simulink model "asbQuadcopters"  (Simulink 9.1)
settings: Solver=VariableStepAuto  StartTime=0.0  StopTime=TFinal  RelTol=1e-3
values from neighbouring files (symbols this model uses):
  Controller =     [data_set.mat]
  Estimator =     [data_set.mat]
  g = 9.81    [data_set.mat]
  init =     [data_set.mat]
  Sensors =     [data_set.mat]
  takeOffDuration = 1    [data_set.mat]
  Ts = 0.005    [data_set.mat]
  Vehicle =     [data_set.mat]
undefined symbols (not defined in the file or in its folder): DiscIntNeverNeededParam, Discrete, Earth, ft, m, s, sigbuilder_block, Time, WGS84
libraries: simulink x39, aerolibconvert2 x4, ctrlSharedLib x3, sharedtransform x3, aerolibfltsims x2, aerolibutil x2, shared6dof x1, aerolibasang x1, dynamicsLibrary x1, aerolibtransform2 x1, environmentLibrary x1, sharedutil x1
(part 1 of 3)
settings Model: SuppressorTable="22 serialization::archive 11 0 6 0 0 1 8 0 0 0 0 6 0 0 1 0 39 asbQuadcopters/Command/Live Time  Ticks 0 6 0 0 2 8 0 0 0 0 6 41 Simulink:DataType:WarningOverFlowDetected 0 0 0 6 0  0  0 0 0 0 8 20160523 0 0 0 10 57 55 0 1 40 SimulinkFixedPoint:util:Overflowoccurred 0 0 0  0  8 20160523 0 10 57 55 0 1"  LogicAnalyzerSignalOrdering=2e0c0a72-345e-4dc5-9c0e-29032ec30a1e,a96d9f9d-3ef5-4050-b6b8-b8019fd01667,c8d366ad-4d1f-40bd-a54a-09e26b883270,8941bdc4-4fa0-4569-8040-854ce7cb60c2,e7686d44-45c9-4c55-ba5d-06b91bc522a8,a75aae3c-0a7a-4dbc-8a75-97ed30805da8,7c481f21-a942-450d-9b23-3950506eae04,f4ffd508-2ff6-4be3-84ec-4b50dbf29143,1f3924a1-458c-46a2-8b2c-9c14621b8789,e4a67875-028c-4c14-9c8e-409b915de7ac  Creator=DES  LastModifiedBy=DES
settings DataIOCC: SaveFormat=Dataset
settings OptimizationCC: LifeSpan=auto
settings DebuggingCC: UnderspecifiedInitializationDetection=Simplified  MergeDetectMultiDrivingBlocksExec=error  SFUnexpectedBacktrackingDiag=error  SFNoUnconditionalDefaultTransitionDiag=error  SFExecutionAtInitializationDiag=warning
settings HardwareCC: ProdBitPerPointer=64  ProdBitPerSizeT=64  ProdBitPerPtrDiffT=64  ProdLargestAtomicFloat=Float  ProdIntDivRoundTo=Zero  ProdEndianess=LittleEndian  ProdWordSize=64  ProdHWDeviceType=Intel->x86-64 (Windows64)
settings ModelReferenceCC: PropagateSignalLabelsOutOfModel=on
settings CodeAppCC: StateflowObjectComments=off
settings GRTTargetCC: TargetLangStandard=C99 (ISO)  CombineOutputUpdateFcns=on  GRTInterface=off
settings ConfigComp: CovMetricSettings=dwe  CovHtmlReporting=off  CovSaveCumulativeToWorkspaceVar=off  CovSaveSingleToWorkspaceVar=off  CovExternalEMLEnable=on

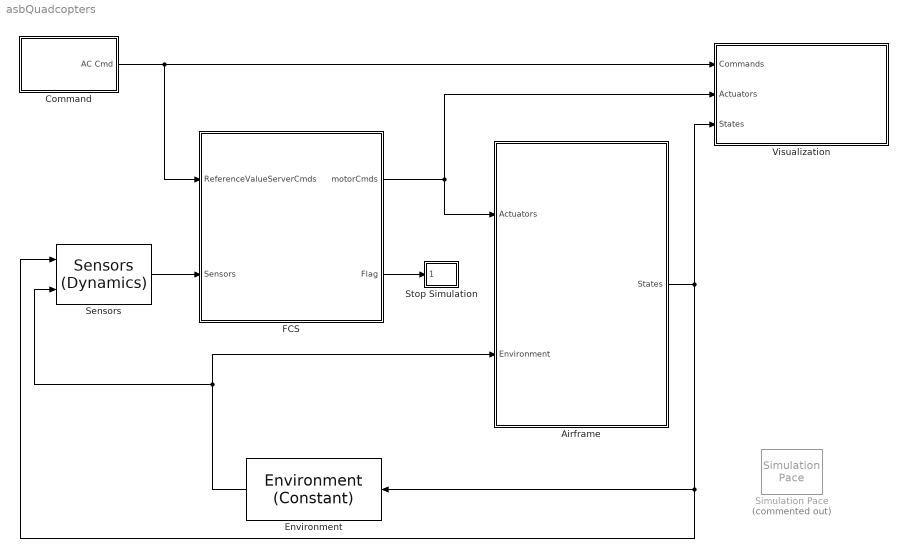
== system asbQuadcopters ==
  Airframe : Subsystem  TreatAsAtomicUnit=on
  Command : Subsystem
  "Environment " : environmentLibrary/Environment (Constant)  VariantControl=VSS_ENVIRONMENT_CST
      settings: SourceProductName=Aerospace Blockset  SourceProductBaseCode=AE
  FCS : Subsystem
  Sensors : sensorsLibrary/Sensors (Dynamics)  SystemSampleTime=-1  VariantControl=VSS_SENSORS_DYNAMICS
      settings: SourceProductName=Aerospace Blockset  SourceProductBaseCode=AE
  Simulation Pace : aerolibanimutils/Simulation Pace  Commented=on  SimulationPace=1  SleepMode=MATLAB Thread  OutputPaceError=off  SampleTime=Ts
      settings: AttributesFormatString=%<SimulationPace> sec/sec
  Stop Simulation : Subsystem
  Visualization : Subsystem
  wires:
  Command/1(AC Cmd) -> Visualization/1(Commands), FCS/1(ReferenceValueServerCmds)
  Sensors/1 -> FCS/2(Sensors)
  Airframe/1(States) -> Visualization/3(States), Sensors/1, "Environment "/1
  "Environment "/1 -> Sensors/2, Airframe/2(Environment)
  FCS/2(Flag) -> Stop Simulation/1(Flags)
  FCS/1(motorCmds) -> Visualization/2(Actuators), Airframe/1(Actuators)

== system asbQuadcopters/Airframe ==
  Actuators : Inport
  Environment : Inport  Port=2
  6DOF (Quaternion) : shared6dof/6DOF (Euler Angles)  units=Metric (MKS)  mtype=Fixed  rep=Euler Angles  xme_0=init.posNED  Vm_0=init.vb  eul_0=init.euler  pm_0=init.angRates  mass_0=Vehicle.Airframe.mass  mass_e=0.5  mass_f=2.0  inertia=Vehicle.Airframe.inertia  inertia_e=eye(3)  inertia_f=2*eye(3)  k_quat=Vehicle.SixDOF.quatGain  vre_flag=on  abi_flag=on  aMode=aMode
      settings: SourceProductBaseCode=AE
  AC model : Subsystem
  Bus setup : Subsystem
  Position on Earth : Subsystem  Priority=1  TreatAsAtomicUnit=on
  Terminator : Terminator
  States : Outport
  wires:
  Actuators/1 -> AC model/1(Actuators)
  Environment/1 -> AC model/2(Environment)
  AC model/1(F_cg) -> 6DOF (Quaternion)/1
  AC model/2(M_cg) -> 6DOF (Quaternion)/2
  6DOF (Quaternion)/1 -> Bus setup/2(V_ned)
  6DOF (Quaternion)/2 -> Position on Earth/1(Xe), Bus setup/3(X_ned)
  6DOF (Quaternion)/3 -> Bus setup/4(Euler)
  6DOF (Quaternion)/6 -> AC model/5(w_b), Bus setup/7(Omega_b)
  6DOF (Quaternion)/7 -> Bus setup/8(dOmega_b)
  6DOF (Quaternion)/9 -> Bus setup/9(Accel_b)
  Bus setup/1(States) -> States/1
  Position on Earth/1(LLA) -> Bus setup/1(LLA)
  6DOF (Quaternion)/5 -> AC model/4(V_b), Bus setup/6(V_b)
  6DOF (Quaternion)/4 -> AC model/3(DCM_be), Bus setup/5(DCM_be)
  6DOF (Quaternion)/8 -> Terminator/1

== system asbQuadcopters/Command ==
  Bus Creator : BusCreator  Inputs=5  OutDataTypeStr=Bus: CommandBus  NonVirtualBus=on
  Clock : Clock
  Compare To Constant : simulink/Logic and Bit Operations/Compare To Constant  relop=<  const=takeOffDuration  OutDataTypeStr=boolean
  Compare To Zero : simulink/Logic and Bit Operations/Compare To Zero  relop===  OutDataTypeStr=boolean
  Compare To Zero1 : simulink/Logic and Bit Operations/Compare To Zero  relop===  OutDataTypeStr=boolean
  Data Type Conversion1 : DataTypeConversion  OutDataTypeStr=single
  Data Type Conversion3 : DataTypeConversion  OutDataTypeStr=single
  Live Time  Ticks : simulink/Sources/Counter Free-Running  NumBits=32  tsamp=Ts
  Logical Operator : Logic  AllPortsSameDT=off  OutDataTypeStr=boolean
  Mux : Mux  Inputs=3
  Mux1 : Mux  Inputs=3
  Position/Attitude Reference : Subsystem  Tag=STV Subsys  LoadFcn=sigbuilder_block('load');  StartFcn=sigbuilder_block('start');  StopFcn=sigbuilder_block('stop');  ClipboardFcn=sigbuilder_block('clipboard');  mask(Sigbuilder block){tuvar=[0:10]}
      mask help: Simulink:masks:SigbuilderBlock_MD
      mask init:
      | if ~strcmp(get_param(bdroot(gcbh),'SimulationStatus'),'stopped') tuvar = sigbuilder_block('maskInit'); end
      settings: CopyFcn=sigbuilder_block('copy');  DeleteFcn=sigbuilder_block('delete');  ModelCloseFcn=sigbuilder_block('modelClose');  PreSaveFcn=sigbuilder_block('preSave');  PauseFcn=sigbuilder_block('pause');  ContinueFcn=sigbuilder_block('continue');  NameChangeFcn=sigbuilder_block('namechange');  OpenFcn=sigbuilder_block('open',[-738.75 224.25 556.5 329.25 ]);  CloseFcn=sigbuilder_block('close');
      mask Display: plot(0, 0, 100, 100,[2, 2, 32, 32, 2], [68, 8, 8, 68, 68],[32, 2], [38, 38], [32, 19, 2],[53, 60, 44], [32, 17, 17, 2],[16, 16, 31, 31]);txt = getActiveGroup(gcbh);text(2, 100, txt,'verticalAlignment', 'top');
  Rate Transition{1..4} (4 alike) : RateTransition  OutPortSampleTime=Ts
  AC Cmd : Outport  OutDataTypeStr=Bus: CommandBus
  wires:
  Bus Creator/1 -> AC Cmd/1
  Position/Attitude Reference/3(Z) -> Mux1/3
  Live Time  Ticks/1 -> Bus Creator/5  "live_time_ticks"
  Position/Attitude Reference/6(Roll) -> Compare To Zero/1, Mux/3  "roll_cmd"
  Position/Attitude Reference/5(Pitch) -> Mux/2, Compare To Zero1/1  "pitch_cmd"
  Compare To Zero1/1 -> Logical Operator/2
  Rate Transition4/1 -> Bus Creator/1  "controlModePosVSOrient"
  Position/Attitude Reference/2(Y) -> Mux1/2
  Rate Transition3/1 -> Bus Creator/3  "takeoff_flag"
  Position/Attitude Reference/4(Yaw) -> Mux/1  "yaw_cmd"
  Data Type Conversion1/1 -> Rate Transition2/1
  Compare To Zero/1 -> Logical Operator/1
  Logical Operator/1 -> Rate Transition4/1
  Mux1/1 -> Data Type Conversion1/1
  Mux/1 -> Data Type Conversion3/1
  Rate Transition2/1 -> Bus Creator/2  "pos_ref"
  Data Type Conversion3/1 -> Rate Transition1/1
  Compare To Constant/1 -> Rate Transition3/1
  Clock/1 -> Compare To Constant/1
  Rate Transition1/1 -> Bus Creator/4  "orient_ref"
  Position/Attitude Reference/1(X) -> Mux1/1

== system asbQuadcopters/FCS ==
  note: Derived from the work by Sertac
      | Karaman and Fabian Riether
  ReferenceValueServerCmds : Inport  OutDataTypeStr=Bus: CommandBus
  Sensors : Inport  Port=2  OutDataTypeStr=Bus: SensorsBus  BusOutputAsStruct=on
  Bus Selector : BusSelector  OutputSignals=controlModePosVSOrient
  Bus Selector1 : BusSelector  OutputSignals=usePosVIS_flag,opticalFlow_data,posVIS_data
  Bus Selector2 : BusSelector  OutputSignals=HAL_acc_SI,HAL_gyro_SI,HAL_ultrasound_SI,HAL_pressure_SI,HAL_vbat_SI
  Bus Selector3 : BusSelector  OutputSignals=HALSensors
  Bus Selector4 : BusSelector  OutputSignals=VisionSensors,SensorCalibration
  Crash Predictor Flags : Subsystem
  Logging : Subsystem  TreatAsAtomicUnit=on
      settings: RTWFcnNameOpts=Use subsystem name
  ReferenceValueServerCmds_1 : InportShadow  OutDataTypeStr=Bus: CommandBus
  Sensors_1 : InportShadow  Port=2  OutDataTypeStr=Bus: SensorsBus  BusOutputAsStruct=on
  Sensors_2 : InportShadow  Port=2  OutDataTypeStr=Bus: SensorsBus  BusOutputAsStruct=on
  State Estimator : Subsystem
  controller : Subsystem
  sensordata_group : Subsystem
  motorCmds : Outport
  Flag : Outport  Port=2
  wires:
  Bus Selector4/2 -> State Estimator/6(sensorCalibration_datin)  "<SensorCalibration>"
  Bus Selector3/1 -> Bus Selector2/1  "<HALSensors>"
  Bus Selector1/3 -> State Estimator/5(posVIS_datin)  "<posVIS_data>"
  Bus Selector/1 -> State Estimator/1(controlModePosVSOrient_flagin)  "<controlModePosVSOrient>"
  Bus Selector2/1 -> sensordata_group/1(HAL_acc_SI)  "<HAL_acc_SI>"
  State Estimator/1(states_estim) -> controller/2(states_estim), Crash Predictor Flags/1(states_estim), Logging/3(states_estim)
  controller/1(motors_refout) -> motorCmds/1, Logging/1(motorCmds)
  Bus Selector2/4 -> sensordata_group/4(HAL_pressure_SI)  "<HAL_pressure_SI>"
  Bus Selector1/1 -> State Estimator/3(usePosVIS_flagin)  "<usePosVIS_flag>"
  sensordata_group/1(sensordata_datin) -> State Estimator/2(sensor_data_in), Logging/6(sensordata_datin)
  Bus Selector1/2 -> State Estimator/4(opticalFlow_datin)  "<opticalFlow_data>"
  ReferenceValueServerCmds/1 -> controller/1(ReferenceValueServerBus), Bus Selector/1
  controller/2(pose_refout) -> Logging/2(posRef)
  Bus Selector4/1 -> Bus Selector1/1  "<VisionSensors>"
  Sensors_1/1 -> Crash Predictor Flags/2(Sensors), Bus Selector4/1
  Bus Selector2/2 -> sensordata_group/2(HAL_gyro_SI)  "<HAL_gyro_SI>"
  Bus Selector2/3 -> sensordata_group/3(HAL_ultrasound_SI)  "<HAL_ultrasound_SI>"
  Sensors/1 -> Bus Selector3/1
  Crash Predictor Flags/1(Flag) -> Flag/1
  Sensors_2/1 -> Logging/5(Sensors)
  Bus Selector2/5 -> sensordata_group/5(HAL_vbat_SI)  "<HAL_vbat_SI>"
  ReferenceValueServerCmds_1/1 -> Logging/4(ReferenceValueServerBus)

== system asbQuadcopters/Stop Simulation ==
  Flags : Inport  OutDataTypeStr=uint8
  Compare To Zero : simulink/Logic and Bit Operations/Compare To Zero  relop=>  OutDataTypeStr=boolean
  Flag has been triggered : Assertion
  Logical Operator : Logic  Operator=NOT  AllPortsSameDT=off  OutDataTypeStr=boolean
  wires:
  Flags/1 -> Compare To Zero/1
  Logical Operator/1 -> Flag has been triggered/1
  Compare To Zero/1 -> Logical Operator/1

== system asbQuadcopters/Visualization ==
  Commands : Inport
  Actuators : Inport  Port=2
  States : Inport  Port=3
  Airspeed Indicator : Subsystem  DialogController=aeroblksHMICreateDDGDialog  DialogControllerArgs=DataTag2  IsWebBlock=on  mask(MWDashboardBlock){webBlockId=18ef8fab-31e9-4f7d-84d7-de450e3677f8, webBlockType=airspeedindicator, ShowLibInBrowser=on, ShowInitialText=on, HMISrcModelName=[]}
      mask prompts: webBlockId "WebBlock Id"; webBlockType "WebBlock Type"; HMISrcModelName "Source Model"
      mask help: aeroblksHMI:aeroblkhmi:AirspeedIndicatorDialogDesc
      mask Help: eval('asbhmihelp(''airspeedindicator'')');
      mask Display:
      | if strcmp(get_param(bdroot(gcb),'BlockDiagramType'), 'library')
      |  image([(matlabroot) '/toolbox/aeroblks/aeroblks/hmi/icons/AirspeedIndicatorIcon.svg'])
      | end
  Altimeter : Subsystem  DialogController=aeroblksHMICreateDDGDialog  DialogControllerArgs=DataTag3  IsWebBlock=on  mask(MWDashboardBlock){webBlockId=100f33d8-dd26-4cf5-9a56-796be033f673, webBlockType=altimeter, ShowLibInBrowser=on, ShowInitialText=on, HMISrcModelName=[]}
      mask prompts: webBlockId "WebBlock Id"; webBlockType "WebBlock Type"; HMISrcModelName "Source Model"
      mask help: aeroblksHMI:aeroblkhmi:AltimeterDialogDesc
      mask Help: eval('asbhmihelp(''altimeter'')');
      mask Display:
      | if strcmp(get_param(bdroot(gcb),'BlockDiagramType'), 'library')
      |  image([(matlabroot) '/toolbox/aeroblks/aeroblks/hmi/icons/AltimeterIcon.svg'])
      | end
  Artificial Horizon : Subsystem  DialogController=aeroblksHMICreateDDGDialog  DialogControllerArgs=DataTag4  IsWebBlock=on  mask(MWDashboardBlock){webBlockId=2f185b59-f257-45c3-93d6-8e4e2ebb9412, webBlockType=artificialhorizon, ShowLibInBrowser=on, ShowInitialText=on, HMISrcModelName=[]}
      mask prompts: webBlockId "WebBlock Id"; webBlockType "WebBlock Type"; HMISrcModelName "Source Model"
      mask help: aeroblksHMI:aeroblkhmi:ArtificialHorizonDialogDesc
      mask Help: eval('asbhmihelp(''artificialhorizon'')');
      mask Display:
      | if strcmp(get_param(bdroot(gcb),'BlockDiagramType'), 'library')
      |  image([(matlabroot) '/toolbox/aeroblks/aeroblks/hmi/icons/ArtificialHorizonIcon.svg'])
      | end
  Climb Rate Indicator : Subsystem  DialogController=aeroblksHMICreateDDGDialog  DialogControllerArgs=DataTag5  IsWebBlock=on  mask(MWDashboardBlock){webBlockId=01b27fea-40d1-4afa-95b8-217bdf758396, webBlockType=climbindicator, ShowLibInBrowser=on, ShowInitialText=on, HMISrcModelName=[]}
      mask prompts: webBlockId "WebBlock Id"; webBlockType "WebBlock Type"; HMISrcModelName "Source Model"
      mask Help: eval('asbhmihelp(''climbindicator'')');
      mask Display:
      | if strcmp(get_param(bdroot(gcb),'BlockDiagramType'), 'library')
      |  image([(matlabroot) '/toolbox/aeroblks/aeroblks/hmi/icons/ClimbIndicatorIcon.svg'])
      | end
  Extract Flight Instruments : Subsystem
  Heading Indicator1 : Subsystem  DialogController=aeroblksHMICreateDDGDialog  DialogControllerArgs=DataTag6  IsWebBlock=on  mask(MWDashboardBlock){webBlockId=349a9895-ae71-4c34-aaf3-8a4b044263fc, webBlockType=headingindicator, ShowLibInBrowser=on, ShowInitialText=on, HMISrcModelName=[]}
      mask prompts: webBlockId "WebBlock Id"; webBlockType "WebBlock Type"; HMISrcModelName "Source Model"
      mask help: aeroblksHMI:aeroblkhmi:HeadingIndicatorDialogDesc
      mask Help: eval('asbhmihelp(''headingindicator'')');
      mask Display:
      | if strcmp(get_param(bdroot(gcb),'BlockDiagramType'), 'library')
      |  image([(matlabroot) '/toolbox/aeroblks/aeroblks/hmi/icons/HeadingIndicatorIcon.svg'])
      | end
  Thruster 1 : Subsystem  DialogController=aeroblksHMICreateDDGDialog  DialogControllerArgs=DataTag7  IsWebBlock=on  mask(MWDashboardBlock){webBlockId=cb5b89b4-9a60-4ffc-8d4b-680aac62b0ad, webBlockType=rpmindicator, ShowLibInBrowser=on, ShowInitialText=on, HMISrcModelName=[]}
      mask prompts: webBlockId "WebBlock Id"; webBlockType "WebBlock Type"; HMISrcModelName "Source Model"
      mask help: aeroblksHMI:aeroblkhmi:RPMIndicatorDialogDesc
      mask Help: eval('asbhmihelp(''rpmindicator'')')
      mask Display:
      | if strcmp(get_param(bdroot(gcb),'BlockDiagramType'), 'library')
      |  image([(matlabroot) '/toolbox/aeroblks/aeroblks/hmi/icons/RPMIndicatorIcon.svg'])
      | end
  Thruster 2 : Subsystem  DialogController=aeroblksHMICreateDDGDialog  DialogControllerArgs=DataTag8  IsWebBlock=on  mask(MWDashboardBlock){webBlockId=f0cf643f-3686-4bab-9794-ec5ca9f0526b, webBlockType=rpmindicator, ShowLibInBrowser=on, ShowInitialText=on, HMISrcModelName=[]}
      mask prompts: webBlockId "WebBlock Id"; webBlockType "WebBlock Type"; HMISrcModelName "Source Model"
      mask help: aeroblksHMI:aeroblkhmi:RPMIndicatorDialogDesc
      mask Help: eval('asbhmihelp(''rpmindicator'')')
      mask Display:
      | if strcmp(get_param(bdroot(gcb),'BlockDiagramType'), 'library')
      |  image([(matlabroot) '/toolbox/aeroblks/aeroblks/hmi/icons/RPMIndicatorIcon.svg'])
      | end
  Thruster 3 : Subsystem  DialogController=aeroblksHMICreateDDGDialog  DialogControllerArgs=DataTag9  IsWebBlock=on  mask(MWDashboardBlock){webBlockId=fde82f48-64f7-4e22-ac0c-568ccc998d28, webBlockType=rpmindicator, ShowLibInBrowser=on, ShowInitialText=on, HMISrcModelName=[]}
      mask prompts: webBlockId "WebBlock Id"; webBlockType "WebBlock Type"; HMISrcModelName "Source Model"
      mask help: aeroblksHMI:aeroblkhmi:RPMIndicatorDialogDesc
      mask Help: eval('asbhmihelp(''rpmindicator'')')
      mask Display:
      | if strcmp(get_param(bdroot(gcb),'BlockDiagramType'), 'library')
      |  image([(matlabroot) '/toolbox/aeroblks/aeroblks/hmi/icons/RPMIndicatorIcon.svg'])
      | end
  Thruster 4 : Subsystem  DialogController=aeroblksHMICreateDDGDialog  DialogControllerArgs=DataTag10  IsWebBlock=on  mask(MWDashboardBlock){webBlockId=9efa2ed4-730f-4ead-a19e-56fcb1fb4e55, webBlockType=rpmindicator, ShowLibInBrowser=on, ShowInitialText=on, HMISrcModelName=[]}
      mask prompts: webBlockId "WebBlock Id"; webBlockType "WebBlock Type"; HMISrcModelName "Source Model"
      mask help: aeroblksHMI:aeroblkhmi:RPMIndicatorDialogDesc
      mask Help: eval('asbhmihelp(''rpmindicator'')')
      mask Display:
      | if strcmp(get_param(bdroot(gcb),'BlockDiagramType'), 'library')
      |  image([(matlabroot) '/toolbox/aeroblks/aeroblks/hmi/icons/RPMIndicatorIcon.svg'])
      | end
  Visualization : Subsystem  Variant=on
  wires:
  Actuators/1 -> Extract Flight Instruments/1(Actuators), Visualization/3(Actuators)
  States/1 -> Visualization/1(States), Extract Flight Instruments/2(States)
  Commands/1 -> Visualization/2(Commands)

== system asbQuadcopters/Airframe/AC model ==
  Actuators : Inport
  Environment : Inport  Port=2
  DCM_be : Inport  Port=3
  V_b : Inport  Port=4  Unit=m/s
  w_b : Inport  Port=5  Unit=rad/s
  Applied Force Calculation : Subsystem
  Bus Selector : BusSelector  OutputSignals=Gravity_ned,AtmosphereBus.air_density
  Drag Calculation : Subsystem
  Gravity Force Calculation : Subsystem
  Motor Forces and Torques : Subsystem
  F_cg : Outport  Unit=N
  M_cg : Outport  Port=2  Unit=N*m
  wires:
  Applied Force Calculation/1(External Forces) -> F_cg/1
  Motor Forces and Torques/2(Motor Torques) -> M_cg/1
  Motor Forces and Torques/1(Motor Forces) -> Applied Force Calculation/3(Motor Forces)
  Bus Selector/1 -> Gravity Force Calculation/2(gravity)  "<Gravity_ned>"
  Gravity Force Calculation/1(gravity force) -> Applied Force Calculation/1(gravity force)
  Environment/1 -> Bus Selector/1
  Bus Selector/2 -> Motor Forces and Torques/2(Density), Drag Calculation/1(Density)  "<air_density>"
  DCM_be/1 -> Gravity Force Calculation/1(DCMbe)
  V_b/1 -> Motor Forces and Torques/1(Vb), Drag Calculation/2(Vb)
  Drag Calculation/1(Drag) -> Applied Force Calculation/2(Aerodynamic Forces)
  Actuators/1 -> Motor Forces and Torques/4(Motor  Commands)
  w_b/1 -> Motor Forces and Torques/3(pqr)

== system asbQuadcopters/Airframe/Bus setup ==
  LLA : Inport  PortDimensions=3
  V_ned : Inport  Port=2  Unit=m/second  PortDimensions=3
  X_ned : Inport  Port=3  Unit=m  PortDimensions=3
  Euler : Inport  Port=4  Unit=rad  PortDimensions=3
  DCM_be : Inport  Port=5  PortDimensions=[3 3]
  V_b : Inport  Port=6  Unit=m/s  PortDimensions=3
  Omega_b : Inport  Port=7  Unit=rad/s  PortDimensions=3
  dOmega_b : Inport  Port=8  Unit=rad/s^2  PortDimensions=3
  Accel_b : Inport  Port=9  Unit=m/s^2  PortDimensions=3
  Bus Creator5 : BusCreator  Inputs=9  OutDataTypeStr=Bus: StatesBus  NonVirtualBus=on
  States : Outport
  wires:
  Bus Creator5/1 -> States/1
  V_b/1 -> Bus Creator5/1  "V_body"
  Omega_b/1 -> Bus Creator5/2  "Omega_body"
  Euler/1 -> Bus Creator5/3  "Euler"
  X_ned/1 -> Bus Creator5/7  "X_ned"
  Accel_b/1 -> Bus Creator5/4  "Accel_body"
  LLA/1 -> Bus Creator5/8  "LLA"
  dOmega_b/1 -> Bus Creator5/5  "dOmega_body"
  DCM_be/1 -> Bus Creator5/9  "DCM_be"
  V_ned/1 -> Bus Creator5/6  "V_ned"

== system asbQuadcopters/Airframe/Position on Earth ==
  Xe : Inport  Unit=m
  Flat Earth to LLA : aerolibtransform2/Flat Earth to LLA  units=Metric (MKS)  ptype=Earth (WGS84)  F=1/298.257223563  R=6378137  LL0=init.posLLA(1:2)  psi=Vehicle.PositionOnEarth.FlatEarthToLLA.xAxis
  Mux : Mux  Inputs=2
  href : Constant  Value=Vehicle.PositionOnEarth.href
  LLA : Outport
  wires:
  Mux/1 -> LLA/1
  Xe/1 -> Flat Earth to LLA/1
  Flat Earth to LLA/1 -> Mux/1
  Flat Earth to LLA/2 -> Mux/2
  href/1 -> Flat Earth to LLA/2

== system asbQuadcopters/Command/Position/Attitude Reference ==
  Demux : Demux  Tag=STV Demux  Outputs=6
  FromWs : FromWorkspace  Tag=STV FromWs  VariableName=tuvar  SampleTime=0  SigBuilderData=DataTag0  VnvData=DataTag1
      SigBuilderData=|
      | common.afterFinalStr = 'Extrapolate'
      | common.sampleTime = 0
      | dataSet.timeRange = [0 100]
      | dataSet.name = 'Group 1'
      | sbobj.Groups.Name = 'Group 1'
      | sbobj.Groups.Signals(1).Name = 'X'
      | sbobj.Groups.Signals(1).XData = [0 100]
      | sbobj.Groups.Signals(1).YData = [0 0]
      | sbobj.Groups.Signals(2).Name = 'Y'
      | sbobj.Groups.Signals(2).XData = [0 100]
      | sbobj.Groups.Signals(2).YData = [0 0]
      | sbobj.Groups.Signals(3).Name = 'Z'
      | sbobj.Groups.Signals(3).XData = [0 1 1 100]
      | sbobj.Groups.Signals(3).YData = [0 0 -1.5 -1.5]
      | sbobj.Groups.Signals(4).Name = 'Yaw'
      | sbobj.Groups.Signals(4).XData = [0 5.5 8 100]
      | sbobj.Groups.Signals(4).YData = [0 0 0 0]
      | sbobj.Groups.Signals(5).Name = 'Pitch'
      | sbobj.Groups.Signals(5).XData = [0 3 4 100]
      | sbobj.Groups.Signals(5).YData = [0 0 0 0]
      | sbobj.Groups.Signals(6).Name = 'Roll'
      | sbobj.Groups.Signals(6).XData = [0 100]
      | sbobj.Groups.Signals(6).YData = [0 0]
      | sbobj.Groups.TimeRange = [0 100]
  X : Outport  Tag=STV Outport
  Y : Outport  Tag=STV Outport  Port=2
  Z : Outport  Tag=STV Outport  Port=3
  Yaw : Outport  Tag=STV Outport  Port=4
  Pitch : Outport  Tag=STV Outport  Port=5
  Roll : Outport  Tag=STV Outport  Port=6
  wires:
  FromWs/1 -> Demux/1
  Demux/1 -> X/1
  Demux/2 -> Y/1
  Demux/3 -> Z/1
  Demux/4 -> Yaw/1
  Demux/5 -> Pitch/1
  Demux/6 -> Roll/1

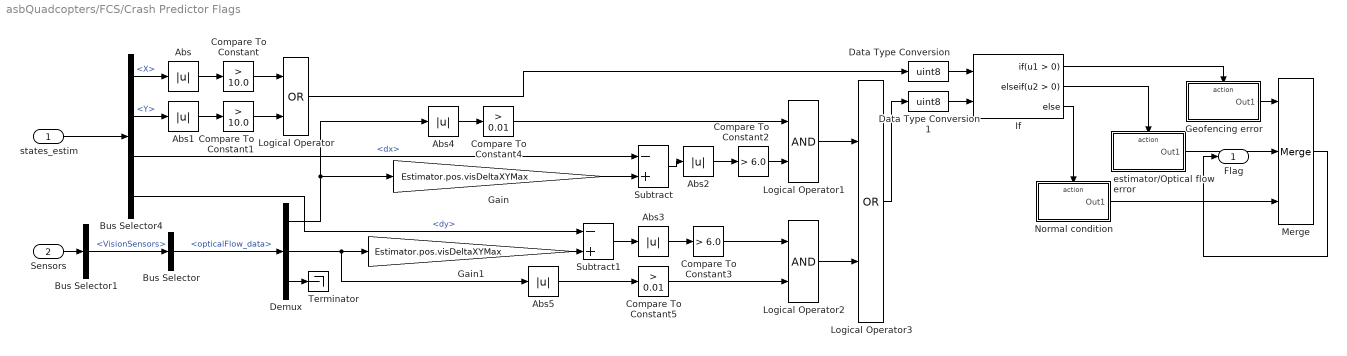
== system asbQuadcopters/FCS/Crash Predictor Flags ==
  states_estim : Inport
  Sensors : Inport  Port=2
  Abs{,1..5} (6 alike) : Abs
  Bus Selector : BusSelector  OutputSignals=opticalFlow_data
  Bus Selector1 : BusSelector  OutputSignals=VisionSensors
  Bus Selector4 : BusSelector  OutputSignals=X,Y,dx,dy
  Compare To Constant : simulink/Logic and Bit Operations/Compare To Constant  relop=>  const=10.0  OutDataTypeStr=boolean
  Compare To Constant1 : simulink/Logic and Bit Operations/Compare To Constant  relop=>  const=10.0  OutDataTypeStr=boolean
  Compare To Constant2 : simulink/Logic and Bit Operations/Compare To Constant  relop=>  const=6.0  OutDataTypeStr=boolean
  Compare To Constant3 : simulink/Logic and Bit Operations/Compare To Constant  relop=>  const=6.0  OutDataTypeStr=boolean
  Compare To Constant4 : simulink/Logic and Bit Operations/Compare To Constant  relop=>  const=0.01  OutDataTypeStr=boolean
  Compare To Constant5 : simulink/Logic and Bit Operations/Compare To Constant  relop=>  const=0.01  OutDataTypeStr=boolean
  Data Type Conversion : DataTypeConversion  OutDataTypeStr=uint8  RndMeth=Nearest
  Data Type Conversion1 : DataTypeConversion  OutDataTypeStr=uint8  RndMeth=Nearest
  Demux : Demux  Outputs=3
  Gain : Gain  Gain=Estimator.pos.visDeltaXYMax
  Gain1 : Gain  Gain=Estimator.pos.visDeltaXYMax
  Geofencing error : Subsystem  TreatAsAtomicUnit=on
  If : If  NumInputs=2  ElseIfExpressions=u2 > 0
  Logical Operator : Logic  Operator=OR  AllPortsSameDT=off
  Logical Operator1 : Logic  AllPortsSameDT=off  OutDataTypeStr=boolean
  Logical Operator2 : Logic  AllPortsSameDT=off  OutDataTypeStr=boolean
  Logical Operator3 : Logic  Operator=OR  AllPortsSameDT=off
  Merge : Merge  Inputs=3  InitialOutput=0
  Normal condition : Subsystem  TreatAsAtomicUnit=on
  Subtract : Sum  Inputs=-+
  Subtract1 : Sum  Inputs=-+
  Terminator : Terminator
  estimator/Optical flow error : Subsystem  TreatAsAtomicUnit=on
  Flag : Outport
  wires:
  Bus Selector4/1 -> Abs/1  "<X>"
  states_estim/1 -> Bus Selector4/1
  Bus Selector4/2 -> Abs1/1  "<Y>"
  Compare To Constant/1 -> Logical Operator/1
  Compare To Constant1/1 -> Logical Operator/2
  Abs/1 -> Compare To Constant/1
  Abs1/1 -> Compare To Constant1/1
  Logical Operator/1 -> Data Type Conversion/1
  Bus Selector/1 -> Demux/1  "<opticalFlow_data>"
  Demux/1 -> Abs4/1, Gain/1
  Demux/2 -> Gain1/1, Abs5/1
  Bus Selector4/3 -> Subtract/1  "<dx>"
  Subtract/1 -> Abs2/1
  Subtract1/1 -> Abs3/1
  Abs2/1 -> Compare To Constant2/1
  Abs3/1 -> Compare To Constant3/1
  Compare To Constant5/1 -> Logical Operator2/2
  Abs4/1 -> Compare To Constant4/1
  Abs5/1 -> Compare To Constant5/1
  Compare To Constant3/1 -> Logical Operator2/1
  Logical Operator1/1 -> Logical Operator3/1
  Logical Operator2/1 -> Logical Operator3/2
  Logical Operator3/1 -> Data Type Conversion1/1
  Demux/3 -> Terminator/1
  Gain/1 -> Subtract/2
  Bus Selector4/4 -> Subtract1/1  "<dy>"
  Gain1/1 -> Subtract1/2
  Compare To Constant4/1 -> Logical Operator1/1
  Compare To Constant2/1 -> Logical Operator1/2
  Sensors/1 -> Bus Selector1/1
  Bus Selector1/1 -> Bus Selector/1  "<VisionSensors>"
  Merge/1 -> Flag/1
  If/1 -> Geofencing error/Action
  If/2 -> estimator/Optical flow error/Action
  If/3 -> Normal condition/Action
  Geofencing error/1(Out1) -> Merge/1
  estimator/Optical flow error/1(Out1) -> Merge/2
  Normal condition/1(Out1) -> Merge/3
  Data Type Conversion/1 -> If/1
  Data Type Conversion1/1 -> If/2

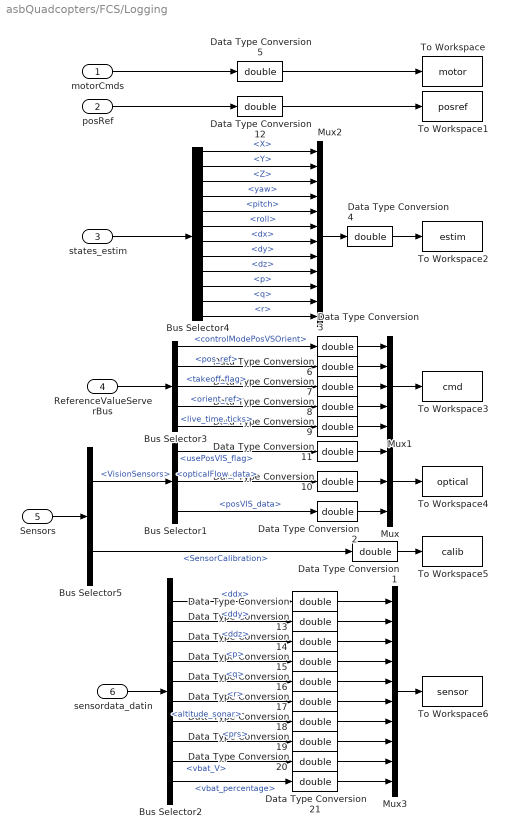
== system asbQuadcopters/FCS/Logging ==
  motorCmds : Inport
  posRef : Inport  Port=2
  states_estim : Inport  Port=3  OutDataTypeStr=Bus: statesEstim_t  BusOutputAsStruct=on
  ReferenceValueServerBus : Inport  Port=4  OutDataTypeStr=Bus: CommandBus  BusOutputAsStruct=on
  Sensors : Inport  Port=5  OutDataTypeStr=Bus: SensorsBus
  sensordata_datin : Inport  Port=6  OutDataTypeStr=Bus: sensordata_t
  Bus Selector1 : BusSelector  OutputSignals=usePosVIS_flag,opticalFlow_data,posVIS_data
  Bus Selector2 : BusSelector  OutputSignals=ddx,ddy,ddz,p,q,r,altitude_sonar,prs,vbat_V,vbat_percentage
  Bus Selector3 : BusSelector  OutputSignals=controlModePosVSOrient,pos_ref,takeoff_flag,orient_ref,live_time_ticks
  Bus Selector4 : BusSelector  OutputSignals=X,Y,Z,yaw,pitch,roll,dx,dy,dz,p,q,r
  Bus Selector5 : BusSelector  OutputSignals=VisionSensors,SensorCalibration
  Data Type Conversion{,1..21} (22 alike) : DataTypeConversion  OutDataTypeStr=double
  Mux : Mux  Inputs=3
  Mux1 : Mux  Inputs=5
  Mux2 : Mux  Inputs=12
  Mux3 : Mux  Inputs=10
  To Workspace : ToWorkspace  VariableName=motor  SaveFormat=Structure With Time  SampleTime=-1
  To Workspace1 : ToWorkspace  VariableName=posref  SaveFormat=Structure With Time  SampleTime=-1
  To Workspace2 : ToWorkspace  VariableName=estim  SaveFormat=Structure With Time  SampleTime=-1
  To Workspace3 : ToWorkspace  VariableName=cmd  SaveFormat=Structure With Time  SampleTime=-1
  To Workspace4 : ToWorkspace  VariableName=optical  SaveFormat=Structure With Time  SampleTime=-1
  To Workspace5 : ToWorkspace  VariableName=calib  SaveFormat=Structure With Time  SampleTime=-1
  To Workspace6 : ToWorkspace  VariableName=sensor  SaveFormat=Structure With Time  SampleTime=-1
  wires:
  Bus Selector3/1 -> Data Type Conversion3/1  "<controlModePosVSOrient>"
  Bus Selector3/3 -> Data Type Conversion7/1  "<takeoff_flag>"
  Bus Selector3/4 -> Data Type Conversion8/1  "<orient_ref>"
  Bus Selector3/5 -> Data Type Conversion9/1  "<live_time_ticks>"
  ReferenceValueServerBus/1 -> Bus Selector3/1
  Bus Selector3/2 -> Data Type Conversion6/1  "<pos_ref>"
  sensordata_datin/1 -> Bus Selector2/1
  Bus Selector2/1 -> Data Type Conversion/1  "<ddx>"
  Sensors/1 -> Bus Selector5/1
  Bus Selector1/1 -> Data Type Conversion11/1  "<usePosVIS_flag>"
  Bus Selector1/2 -> Data Type Conversion10/1  "<opticalFlow_data>"
  Bus Selector1/3 -> Data Type Conversion2/1  "<posVIS_data>"
  Data Type Conversion1/1 -> To Workspace5/1
  Bus Selector5/2 -> Data Type Conversion1/1  "<SensorCalibration>"
  Mux/1 -> To Workspace4/1
  Data Type Conversion4/1 -> To Workspace2/1
  motorCmds/1 -> Data Type Conversion5/1
  Data Type Conversion5/1 -> To Workspace/1
  Mux1/1 -> To Workspace3/1
  states_estim/1 -> Bus Selector4/1
  Mux2/1 -> Data Type Conversion4/1
  Bus Selector4/4 -> Mux2/4  "<yaw>"
  Bus Selector4/6 -> Mux2/6  "<roll>"
  Bus Selector4/5 -> Mux2/5  "<pitch>"
  Bus Selector4/9 -> Mux2/9  "<dz>"
  Bus Selector4/7 -> Mux2/7  "<dx>"
  Bus Selector4/8 -> Mux2/8  "<dy>"
  Bus Selector4/10 -> Mux2/10  "<p>"
  Bus Selector4/12 -> Mux2/12  "<r>"
  Bus Selector4/2 -> Mux2/2  "<Y>"
  Bus Selector4/11 -> Mux2/11  "<q>"
  Bus Selector4/3 -> Mux2/3  "<Z>"
  Bus Selector4/1 -> Mux2/1  "<X>"
  Data Type Conversion3/1 -> Mux1/1
  Data Type Conversion6/1 -> Mux1/2
  Data Type Conversion7/1 -> Mux1/3
  Data Type Conversion8/1 -> Mux1/4
  Data Type Conversion9/1 -> Mux1/5
  Data Type Conversion2/1 -> Mux/3
  Data Type Conversion10/1 -> Mux/2
  Data Type Conversion11/1 -> Mux/1
  posRef/1 -> Data Type Conversion12/1
  Data Type Conversion12/1 -> To Workspace1/1
  Bus Selector2/2 -> Data Type Conversion13/1  "<ddy>"
  Bus Selector2/3 -> Data Type Conversion14/1  "<ddz>"
  Bus Selector2/4 -> Data Type Conversion15/1  "<p>"
  Bus Selector2/5 -> Data Type Conversion16/1  "<q>"
  Bus Selector2/6 -> Data Type Conversion17/1  "<r>"
  Bus Selector2/7 -> Data Type Conversion18/1  "<altitude_sonar>"
  Bus Selector2/8 -> Data Type Conversion19/1  "<prs>"
  Bus Selector2/9 -> Data Type Conversion20/1  "<vbat_V>"
  Bus Selector2/10 -> Data Type Conversion21/1  "<vbat_percentage>"
  Data Type Conversion/1 -> Mux3/1
  Data Type Conversion13/1 -> Mux3/2
  Data Type Conversion14/1 -> Mux3/3
  Data Type Conversion15/1 -> Mux3/4
  Data Type Conversion16/1 -> Mux3/5
  Data Type Conversion17/1 -> Mux3/6
  Data Type Conversion18/1 -> Mux3/7
  Data Type Conversion19/1 -> Mux3/8
  Data Type Conversion20/1 -> Mux3/9
  Data Type Conversion21/1 -> Mux3/10
  Mux3/1 -> To Workspace6/1
  Bus Selector5/1 -> Bus Selector1/1  "<VisionSensors>"

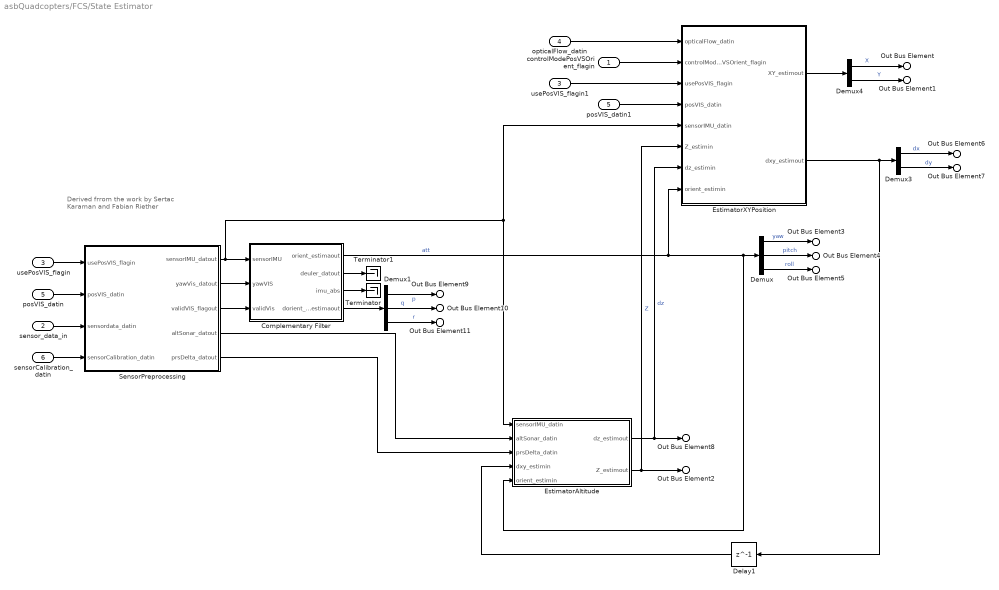
== system asbQuadcopters/FCS/State Estimator ==
  note: Derived frrom the work by Sertac
      | Karaman and Fabian Riether
  controlModePosVSOrient_flagin : Inport  OutDataTypeStr=boolean
  sensor_data_in : Inport  Port=2
  usePosVIS_flagin : Inport  Port=3
  opticalFlow_datin : Inport  Port=4
  posVIS_datin : Inport  Port=5
  sensorCalibration_datin : Inport  Port=6
  Complementary Filter : Subsystem
  Delay1 : Delay  DelayLength=1  InitialCondition=0
  Demux : Demux  Outputs=3
  Demux1 : Demux  Outputs=3
  Demux3 : Demux  Outputs=2
  Demux4 : Demux  Outputs=2
  EstimatorAltitude : Subsystem
  EstimatorXYPosition : Subsystem
  SensorPreprocessing : Subsystem
  Terminator : Terminator
  Terminator1 : Terminator
  posVIS_datin1 : InportShadow  Port=5
  usePosVIS_flagin1 : InportShadow  Port=3
  Out Bus Element : Outport  PortName=states_estim  Element=X
  Out Bus Element1 : Outport  PortName=states_estim  Element=Y
  Out Bus Element2 : Outport  PortName=states_estim  Element=Z
  Out Bus Element3 : Outport  PortName=states_estim  Element=yaw
  Out Bus Element4 : Outport  PortName=states_estim  Element=pitch
  Out Bus Element5 : Outport  PortName=states_estim  Element=roll
  Out Bus Element6 : Outport  PortName=states_estim  Element=dx
  Out Bus Element7 : Outport  PortName=states_estim  Element=dy
  Out Bus Element8 : Outport  PortName=states_estim  Element=dz
  Out Bus Element9 : Outport  PortName=states_estim  Element=p
  Out Bus Element10 : Outport  PortName=states_estim  Element=q
  Out Bus Element11 : Outport  PortName=states_estim  Element=r
  wires:
  EstimatorXYPosition/2(dxy_estimout) -> Delay1/1, Demux3/1
  posVIS_datin/1 -> SensorPreprocessing/2(posVIS_datin)
  Demux1/3 -> Out Bus Element11/1  "r"
  Demux/3 -> Out Bus Element5/1  "roll"
  Demux4/2 -> Out Bus Element1/1  "Y"
  EstimatorXYPosition/1(XY_estimout) -> Demux4/1
  Complementary Filter/2(deuler_datout) -> Terminator1/1
  Complementary Filter/4(dorient_estimaout) -> Demux1/1
  SensorPreprocessing/3(validVIS_flagout) -> Complementary Filter/3(validVis)
  sensor_data_in/1 -> SensorPreprocessing/3(sensordata_datin)
  opticalFlow_datin/1 -> EstimatorXYPosition/1(opticalFlow_datin)
  Demux4/1 -> Out Bus Element/1  "X"
  SensorPreprocessing/1(sensorIMU_datout) -> Complementary Filter/1(sensorIMU), EstimatorAltitude/1(sensorIMU_datin), EstimatorXYPosition/5(sensorIMU_datin)
  SensorPreprocessing/5(prsDelta_datout) -> EstimatorAltitude/3(prsDelta_datin)
  Demux3/2 -> Out Bus Element7/1  "dy"
  SensorPreprocessing/2(yawVis_datout) -> Complementary Filter/2(yawVIS)
  SensorPreprocessing/4(altSonar_datout) -> EstimatorAltitude/2(altSonar_datin)
  usePosVIS_flagin/1 -> SensorPreprocessing/1(usePosVIS_flagin)
  EstimatorAltitude/1(dz_estimout) -> Out Bus Element8/1, EstimatorXYPosition/7(dz_estimin)  "dz"
  EstimatorAltitude/2(Z_estimout) -> Out Bus Element2/1, EstimatorXYPosition/6(Z_estimin)  "Z"
  Demux1/1 -> Out Bus Element9/1  "p"
  Demux3/1 -> Out Bus Element6/1  "dx"
  Complementary Filter/3(imu_abs) -> Terminator/1
  Demux/2 -> Out Bus Element4/1  "pitch"
  controlModePosVSOrient_flagin/1 -> EstimatorXYPosition/2(controlModePosVSOrient_flagin)
  Complementary Filter/1(orient_estimaout) -> EstimatorAltitude/5(orient_estimin), Demux/1, EstimatorXYPosition/8(orient_estimin)  "att"
  Demux/1 -> Out Bus Element3/1  "yaw"
  Delay1/1 -> EstimatorAltitude/4(dxy_estimin)
  Demux1/2 -> Out Bus Element10/1  "q"
  usePosVIS_flagin1/1 -> EstimatorXYPosition/3(usePosVIS_flagin)
  posVIS_datin1/1 -> EstimatorXYPosition/4(posVIS_datin)
  sensorCalibration_datin/1 -> SensorPreprocessing/4(sensorCalibration_datin)

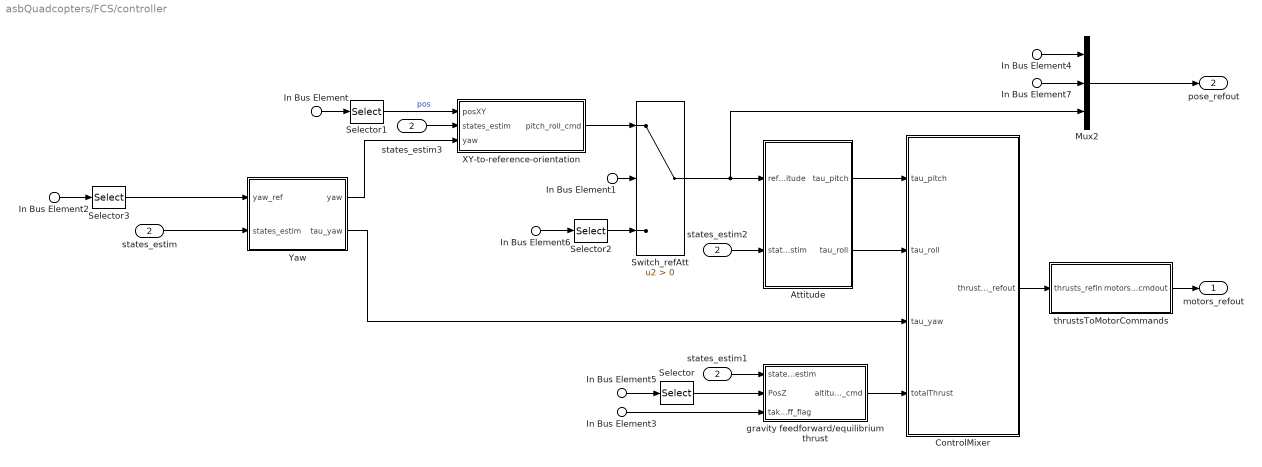
== system asbQuadcopters/FCS/controller ==
  In Bus Element1 : Inport  PortName=ReferenceValueServerBus  Element=controlModePosVSOrient
  In Bus Element : Inport  PortName=ReferenceValueServerBus  Element=pos_ref
  In Bus Element4 : Inport  PortName=ReferenceValueServerBus  Element=pos_ref
  In Bus Element5 : Inport  PortName=ReferenceValueServerBus  Element=pos_ref
  In Bus Element2 : Inport  PortName=ReferenceValueServerBus  Element=orient_ref
  In Bus Element6 : Inport  PortName=ReferenceValueServerBus  Element=orient_ref
  In Bus Element7 : Inport  PortName=ReferenceValueServerBus  Element=orient_ref
  In Bus Element3 : Inport  PortName=ReferenceValueServerBus  Element=takeoff_flag
  states_estim : Inport  Port=2
  Attitude : Subsystem
  ControlMixer : Subsystem
  Mux2 : Mux  Inputs=3
  Selector : Selector  InputPortWidth=3  IndexOptions=Index vector (dialog)  Indices=3  OutputSizes=1
  Selector1 : Selector  InputPortWidth=3  IndexOptions=Index vector (dialog)  Indices=[1 2]  OutputSizes=1
  Selector2 : Selector  InputPortWidth=3  IndexOptions=Index vector (dialog)  Indices=[2 3]  OutputSizes=1
  Selector3 : Selector  InputPortWidth=3  IndexOptions=Index vector (dialog)  Indices=1  OutputSizes=1
  Switch_refAtt : Switch  Criteria=u2 > Threshold
  XY-to-reference-orientation : Subsystem
  Yaw : Subsystem
  gravity feedforward/equilibrium thrust : Subsystem
  states_estim1 : InportShadow  Port=2
  states_estim2 : InportShadow  Port=2
  states_estim3 : InportShadow  Port=2
  thrustsToMotorCommands : Subsystem
  motors_refout : Outport
  pose_refout : Outport  Port=2
  wires:
  thrustsToMotorCommands/1(motors_cmdout) -> motors_refout/1
  In Bus Element1/1 -> Switch_refAtt/2
  XY-to-reference-orientation/1(pitch_roll_cmd) -> Switch_refAtt/1
  In Bus Element2/1 -> Selector3/1
  In Bus Element/1 -> Selector1/1
  Selector3/1 -> Yaw/1(yaw_ref)
  Selector1/1 -> XY-to-reference-orientation/1(posXY)  "pos"
  ControlMixer/1(thrusts_refout) -> thrustsToMotorCommands/1(thrusts_refin)
  In Bus Element3/1 -> gravity feedforward/equilibrium thrust/3(takeoff_flag)
  states_estim/1 -> Yaw/2(states_estim)
  Switch_refAtt/1 -> Attitude/1(refAttitude), Mux2/3
  Yaw/1(yaw) -> XY-to-reference-orientation/3(yaw)
  gravity feedforward/equilibrium thrust/1(altitude_cmd) -> ControlMixer/4(totalThrust)
  Mux2/1 -> pose_refout/1
  Attitude/1(tau_pitch) -> ControlMixer/1(tau_pitch)
  Attitude/2(tau_roll) -> ControlMixer/2(tau_roll)
  Yaw/2(tau_yaw) -> ControlMixer/3(tau_yaw)
  states_estim1/1 -> gravity feedforward/equilibrium thrust/1(states_estim)
  states_estim2/1 -> Attitude/2(states_estim)
  states_estim3/1 -> XY-to-reference-orientation/2(states_estim)
  In Bus Element4/1 -> Mux2/1
  Selector/1 -> gravity feedforward/equilibrium thrust/2(PosZ)
  In Bus Element5/1 -> Selector/1
  In Bus Element6/1 -> Selector2/1
  Selector2/1 -> Switch_refAtt/3
  In Bus Element7/1 -> Mux2/2

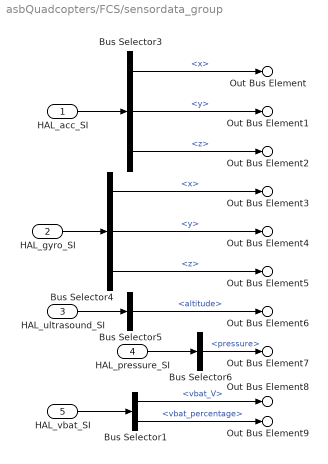
== system asbQuadcopters/FCS/sensordata_group ==
  HAL_acc_SI : Inport  OutDataTypeStr=Bus: HAL_acc_SI_t
  HAL_gyro_SI : Inport  Port=2  OutDataTypeStr=Bus: HAL_gyro_SI_t
  HAL_ultrasound_SI : Inport  Port=3  OutDataTypeStr=Bus: HAL_ultrasound_SI_t
  HAL_pressure_SI : Inport  Port=4  OutDataTypeStr=Bus: HAL_pressure_SI_t
  HAL_vbat_SI : Inport  Port=5  OutDataTypeStr=Bus: HAL_vbat_SI_t
  Bus Selector1 : BusSelector  OutputSignals=vbat_V,vbat_percentage
  Bus Selector3 : BusSelector  OutputSignals=x,y,z
  Bus Selector4 : BusSelector  OutputSignals=x,y,z
  Bus Selector5 : BusSelector  OutputSignals=altitude
  Bus Selector6 : BusSelector  OutputSignals=pressure
  Out Bus Element : Outport  PortName=sensordata_datin  Element=ddx
  Out Bus Element1 : Outport  PortName=sensordata_datin  Element=ddy
  Out Bus Element2 : Outport  PortName=sensordata_datin  Element=ddz
  Out Bus Element3 : Outport  PortName=sensordata_datin  Element=p
  Out Bus Element4 : Outport  PortName=sensordata_datin  Element=q
  Out Bus Element5 : Outport  PortName=sensordata_datin  Element=r
  Out Bus Element6 : Outport  PortName=sensordata_datin  Element=altitude_sonar
  Out Bus Element7 : Outport  PortName=sensordata_datin  Element=prs
  Out Bus Element8 : Outport  PortName=sensordata_datin  Element=vbat_V
  Out Bus Element9 : Outport  PortName=sensordata_datin  Element=vbat_percentage
  wires:
  HAL_gyro_SI/1 -> Bus Selector4/1
  HAL_acc_SI/1 -> Bus Selector3/1
  HAL_pressure_SI/1 -> Bus Selector6/1
  HAL_ultrasound_SI/1 -> Bus Selector5/1
  Bus Selector4/1 -> Out Bus Element3/1  "<x>"
  Bus Selector3/3 -> Out Bus Element2/1  "<z>"
  Bus Selector4/3 -> Out Bus Element5/1  "<z>"
  Bus Selector5/1 -> Out Bus Element6/1  "<altitude>"
  Bus Selector6/1 -> Out Bus Element7/1  "<pressure>"
  Bus Selector4/2 -> Out Bus Element4/1  "<y>"
  Bus Selector3/1 -> Out Bus Element/1  "<x>"
  Bus Selector3/2 -> Out Bus Element1/1  "<y>"
  Bus Selector1/1 -> Out Bus Element8/1  "<vbat_V>"
  HAL_vbat_SI/1 -> Bus Selector1/1
  Bus Selector1/2 -> Out Bus Element9/1  "<vbat_percentage>"

== system asbQuadcopters/Visualization/Airspeed Indicator ==

== system asbQuadcopters/Visualization/Altimeter ==

== system asbQuadcopters/Visualization/Artificial Horizon ==

== system asbQuadcopters/Visualization/Climb Rate Indicator ==

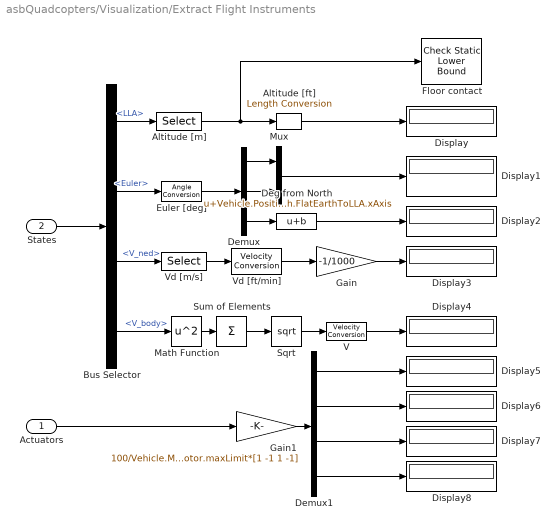
== system asbQuadcopters/Visualization/Extract Flight Instruments ==
  Actuators : Inport
  States : Inport  Port=2
  Altitude [ft] : aerolibconvert2/Length Conversion  IU=m  OU=ft
  Altitude [m] : Selector  InputPortWidth=3  IndexOptions=Index vector (dialog)  Indices=[3]  OutputSizes=1
  Bus Selector : BusSelector  OutputSignals=LLA,Euler,V_ned,V_body
  Deg from North : Bias  Bias=Vehicle.PositionOnEarth.FlatEarthToLLA.xAxis
  Demux : Demux  Outputs=3
  Demux1 : Demux
  Display{,1..8} (9 alike) : Display
  Euler [deg] : aerolibconvert2/Angle Conversion  IU=rad  OU=deg
  Floor contact : simulink/Model Verification/Check Static  Lower Bound  Description=init.posLLA(3) <= u  min=init.posLLA(3)  min_included=on  enabled=on  stopWhenAssertionFail=on  export=off  icon=graphic
      settings: SourceProductName=Simulink
  Gain : Gain  Gain=-1/1000
  Gain1 : Gain  Gain=100/Vehicle.Motor.maxLimit*[1 -1 1 -1]
  Math Function : Math  Operator=square  SaturateOnIntegerOverflow=on
  Mux : Mux  Inputs=2
  Sqrt : Sqrt  SaturateOnIntegerOverflow=on
  Sum of Elements : Sum  Inputs=+
  V : aerolibconvert2/Velocity Conversion  IU=m/s  OU=kts
  Vd [ft/min] : aerolibconvert2/Velocity Conversion  IU=m/s  OU=ft/min
  Vd [m/s] : Selector  InputPortWidth=3  IndexOptions=Index vector (dialog)  Indices=[3]  OutputSizes=1
  wires:
  Bus Selector/1 -> Altitude [m]/1  "<LLA>"
  Altitude [m]/1 -> Floor contact/1, Altitude [ft]/1
  States/1 -> Bus Selector/1
  Altitude [ft]/1 -> Display/1
  Bus Selector/2 -> Euler [deg]/1  "<Euler>"
  Euler [deg]/1 -> Demux/1
  Demux/1 -> Mux/1
  Demux/2 -> Mux/2
  Mux/1 -> Display1/1
  Deg from North/1 -> Display2/1
  Bus Selector/3 -> Vd [m/s]/1  "<V_ned>"
  Vd [m/s]/1 -> Vd [ft/min]/1
  Vd [ft/min]/1 -> Gain/1
  Gain/1 -> Display3/1
  Math Function/1 -> Sum of Elements/1
  Sum of Elements/1 -> Sqrt/1
  Bus Selector/4 -> Math Function/1  "<V_body>"
  Sqrt/1 -> V/1
  V/1 -> Display4/1
  Gain1/1 -> Demux1/1
  Demux1/1 -> Display5/1
  Demux1/2 -> Display6/1
  Demux1/3 -> Display7/1
  Demux1/4 -> Display8/1
  Actuators/1 -> Gain1/1
  Demux/3 -> Deg from North/1

== system asbQuadcopters/Visualization/Heading Indicator1 ==

== system asbQuadcopters/Visualization/Thruster 1 ==

== system asbQuadcopters/Visualization/Thruster 2 ==

== system asbQuadcopters/Visualization/Thruster 3 ==

== system asbQuadcopters/Visualization/Thruster 4 ==

== system asbQuadcopters/Visualization/Visualization ==
  note: VSS_VISUALIZATION = 0 will select scopes as means to visualie variables/states
      | VSS_VISUALIZATION = 1 will send select states in a variable to the workspace
      | VSS_VISUALIZATION = 2 will use FlightGear as visualization
      | VSS_VISUALIZATION = 3 will use a Simulink 3D interface
  States : Inport  OutDataTypeStr=Bus: StatesBus
  Commands : Inport  Port=2  OutDataTypeStr=Bus: CommandBus
  Actuators : Inport  Port=3
  FlightGear : Subsystem  VariantControl=VSS_VISUALIZATION_FLIGHTGEAR
      mask init:
      | visualizationFlightGearVars;
  Scopes : Subsystem  VariantControl=VSS_VISUALIZATION_SCOPES
  Simulink 3D : Subsystem  VariantControl=VSS_VISUALIZATION_SL3D
      mask init:
      | visualizationFlightGearVars;
  Workspace : Subsystem  VariantControl=VSS_VISUALIZATION_WORKSPACE

== system asbQuadcopters/Airframe/AC model/Applied Force Calculation ==
  gravity force : Inport  Unit=N
  Aerodynamic Forces : Inport  Port=2  Unit=N
  Motor Forces : Inport  Port=3  Unit=N
  Add1 : Sum  Inputs=+++
  Signal Specification : SignalSpecification  Dimensions=3
  External Forces : Outport  Unit=N
  wires:
  Add1/1 -> Signal Specification/1
  Motor Forces/1 -> Add1/3  "Motor Thrust"
  Aerodynamic Forces/1 -> Add1/2
  gravity force/1 -> Add1/1
  Signal Specification/1 -> External Forces/1

== system asbQuadcopters/Airframe/AC model/Drag Calculation ==
  Density : Inport  Unit=kg/m^3
  Vb : Inport  Port=2  Unit=m/second
  Drag Calc : Subsystem
  Gain3 : Gain  Gain=-1
  Product : Product  RndMeth=Zero
  Sign : Signum  ZeroCross=off
  Drag : Outport  Unit=N
  wires:
  Density/1 -> Drag Calc/1(Density)
  Sign/1 -> Gain3/1
  Drag Calc/1(drag) -> Product/1
  Gain3/1 -> Product/2
  Product/1 -> Drag/1  "xDrag"
  Vb/1 -> Sign/1, Drag Calc/2(vel)

== system asbQuadcopters/Airframe/AC model/Gravity Force Calculation ==
  DCMbe : Inport
  gravity : Inport  Port=2  Unit=m/s^2
  Gain1 : Gain  Gain=Vehicle.Airframe.mass
  Product : Product  Multiplication=Matrix(*)
  gravity force : Outport  Unit=N
  wires:
  gravity/1 -> Gain1/1
  Gain1/1 -> Product/2  "gravity force NED"
  Product/1 -> gravity force/1
  DCMbe/1 -> Product/1

== system asbQuadcopters/Airframe/AC model/Motor Forces and Torques ==
  Vb : Inport
  Density : Inport  Port=2
  pqr : Inport  Port=3
  Motor  Commands : Inport  Port=4
  D1 : Constant  Value=[Vehicle.Airframe.xy -Vehicle.Airframe.xy Vehicle.Airframe.h]
  D2 : Constant  Value=[Vehicle.Airframe.xy Vehicle.Airframe.xy Vehicle.Airframe.h]
  D3 : Constant  Value=[-Vehicle.Airframe.xy Vehicle.Airframe.xy Vehicle.Airframe.h]
  D4 : Constant  Value=[-Vehicle.Airframe.xy -Vehicle.Airframe.xy Vehicle.Airframe.h]
  For Each Subsystem : Subsystem  TreatAsAtomicUnit=on
  MotorsToW : Subsystem
  Sum of Elements : Sum  Inputs=+  CollapseMode=Specified dimension  CollapseDim=2
  Sum of Elements1 : Sum  Inputs=+  CollapseMode=Specified dimension  CollapseDim=2
  Vector Concatenate : Concatenate  NumInputs=4  Mode=Multidimensional array  ConcatenateDimension=2
  Motor Forces : Outport  Unit=N
  Motor Torques : Outport  Port=2  Unit=N*m
  wires:
  D4/1 -> Vector Concatenate/4
  MotorsToW/1(omegas_datout) -> For Each Subsystem/4(w)
  Vector Concatenate/1 -> For Each Subsystem/5(D)
  For Each Subsystem/2(Moments) -> Sum of Elements1/1
  pqr/1 -> For Each Subsystem/3(Omega)
  Vb/1 -> For Each Subsystem/1(Vb)
  Motor  Commands/1 -> MotorsToW/1(motors_datin)
  D1/1 -> Vector Concatenate/1
  D3/1 -> Vector Concatenate/3
  D2/1 -> Vector Concatenate/2
  Sum of Elements1/1 -> Motor Torques/1
  Density/1 -> For Each Subsystem/2(rho)
  Sum of Elements/1 -> Motor Forces/1
  For Each Subsystem/1(Forces) -> Sum of Elements/1

== system asbQuadcopters/FCS/Crash Predictor Flags/Geofencing error ==
  Action Port : ActionPort  ActionType=then
  Constant : Constant  OutDataTypeStr=uint8
  Out1 : Outport
  wires:
  Constant/1 -> Out1/1

== system asbQuadcopters/FCS/Crash Predictor Flags/Normal condition ==
  Action Port : ActionPort  ActionType=else
  Constant : Constant  Value=0  OutDataTypeStr=uint8
  Out1 : Outport
  wires:
  Constant/1 -> Out1/1

== system asbQuadcopters/FCS/Crash Predictor Flags/estimator/Optical flow error ==
  Action Port : ActionPort  ActionType=elseif
  Constant : Constant  Value=99  OutDataTypeStr=uint8
  Out1 : Outport
  wires:
  Constant/1 -> Out1/1

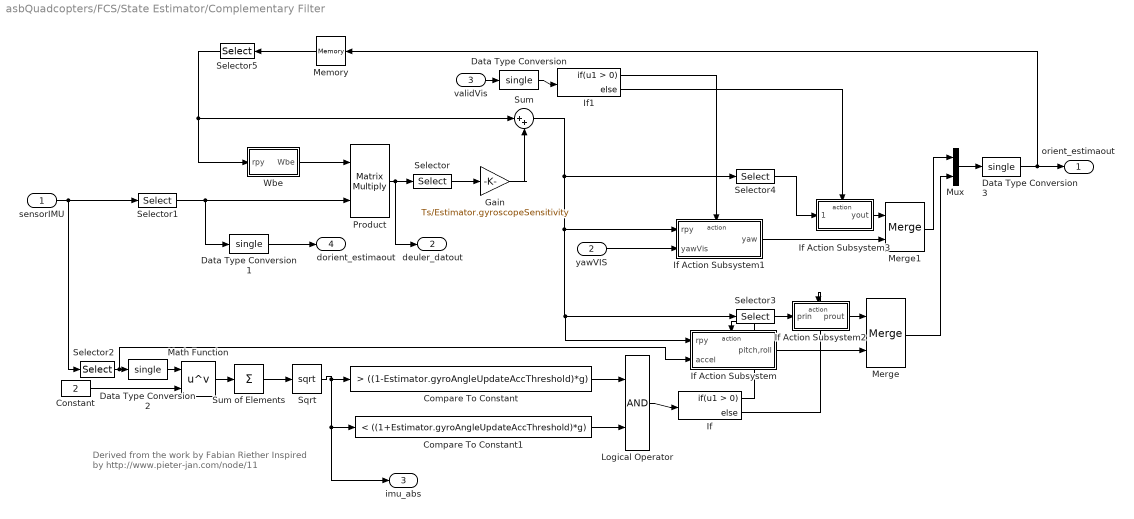
== system asbQuadcopters/FCS/State Estimator/Complementary Filter ==
  note: Derived from the work by Fabian Riether
      | Inspired by http://www.pieter-jan.com/node/11
  sensorIMU : Inport  OutDataTypeStr=single
  yawVIS : Inport  Port=2
  validVis : Inport  Port=3
  Compare To Constant : simulink/Logic and Bit Operations/Compare To Constant  relop=>  const=((1-Estimator.gyroAngleUpdateAccThreshold)*g)  OutDataTypeStr=boolean
  Compare To Constant1 : simulink/Logic and Bit Operations/Compare To Constant  relop=<  const=((1+Estimator.gyroAngleUpdateAccThreshold)*g)  OutDataTypeStr=boolean
  Constant : Constant  Value=2  OutDataTypeStr=single
  Data Type Conversion{,1..3} (4 alike) : DataTypeConversion  OutDataTypeStr=single
  Gain : Gain  Gain=Ts/Estimator.gyroscopeSensitivity
  If : If
  If Action Subsystem : Subsystem  TreatAsAtomicUnit=on
  If Action Subsystem1 : Subsystem  TreatAsAtomicUnit=on
  If Action Subsystem2 : Subsystem  TreatAsAtomicUnit=on
  If Action Subsystem3 : Subsystem  TreatAsAtomicUnit=on
  If1 : If
  Logical Operator : Logic  AllPortsSameDT=off  OutDataTypeStr=fixdt(1,16)
  Math Function : Math  Operator=pow  SaturateOnIntegerOverflow=on
  Memory : Memory  InitialCondition=single(Estimator.complementaryFilterInit)  InheritSampleTime=on
  Merge : Merge
  Merge1 : Merge
  Mux : Mux  Inputs=2
  Product : Product  Multiplication=Matrix(*)
  Selector : Selector  InputPortWidth=3  IndexOptions=Index vector (dialog)  Indices=[3 2 1]  OutputSizes=1
  Selector1 : Selector  InputPortWidth=6  IndexOptions=Index vector (dialog)  Indices=[4 5 6]  OutputSizes=1
  Selector2 : Selector  InputPortWidth=6  IndexOptions=Index vector (dialog)  Indices=[1 2 3]  OutputSizes=1
  Selector3 : Selector  InputPortWidth=3  IndexOptions=Index vector (dialog)  Indices=[2 1]  OutputSizes=1
  Selector4 : Selector  InputPortWidth=3  IndexOptions=Index vector (dialog)  Indices=[3]  OutputSizes=1
  Selector5 : Selector  InputPortWidth=3  IndexOptions=Index vector (dialog)  Indices=[3 2 1]  OutputSizes=1
  Sqrt : Sqrt  SaturateOnIntegerOverflow=on
  Sum : Sum  Inputs=|++
  Sum of Elements : Sum  Inputs=+
  Wbe : Subsystem
  orient_estimaout : Outport
  deuler_datout : Outport  Port=2
  imu_abs : Outport  Port=3  OutDataTypeStr=single
  dorient_estimaout : Outport  Port=4
  wires:
  sensorIMU/1 -> Selector1/1, Selector2/1
  Product/1 -> deuler_datout/1, Selector/1
  Wbe/1(Wbe) -> Product/1
  Selector/1 -> Gain/1
  Gain/1 -> Sum/2
  Memory/1 -> Selector5/1
  Sum of Elements/1 -> Sqrt/1
  Math Function/1 -> Sum of Elements/1
  Constant/1 -> Math Function/2
  Selector2/1 -> If Action Subsystem/2(accel), Data Type Conversion2/1
  Sqrt/1 -> imu_abs/1, Compare To Constant1/1, Compare To Constant/1
  Compare To Constant/1 -> Logical Operator/1
  Compare To Constant1/1 -> Logical Operator/2
  If Action Subsystem/1(pitch,roll) -> Merge/2
  Sum/1 -> If Action Subsystem1/1(rpy), If Action Subsystem/1(rpy), Selector3/1, Selector4/1
  Selector3/1 -> If Action Subsystem2/1(prin)
  yawVIS/1 -> If Action Subsystem1/2(yawVis)
  Selector4/1 -> If Action Subsystem3/1(yawin)
  If Action Subsystem1/1(yaw) -> Merge1/2
  Merge/1 -> Mux/2
  Mux/1 -> Data Type Conversion3/1
  If Action Subsystem2/1(prout) -> Merge/1
  If/2 -> If Action Subsystem2/Action
  If Action Subsystem3/1(yout) -> Merge1/1
  If1/2 -> If Action Subsystem3/Action
  Logical Operator/1 -> If/1
  If/1 -> If Action Subsystem/Action
  If1/1 -> If Action Subsystem1/Action
  Data Type Conversion/1 -> If1/1
  validVis/1 -> Data Type Conversion/1
  Selector1/1 -> Product/2, Data Type Conversion1/1
  Data Type Conversion2/1 -> Math Function/1
  Data Type Conversion3/1 -> Memory/1, orient_estimaout/1
  Merge1/1 -> Mux/1
  Selector5/1 -> Sum/1, Wbe/1(rpy)
  Data Type Conversion1/1 -> dorient_estimaout/1
